simulink model "LD1"  (Simulink 7.9)
settings: Solver=ode3  StartTime=0.0  StopTime=7.0  FixedStep=1e-4  RelTol=1e-3
libraries: dsparch4 x4, simulink x1
settings Model: Creator=user  LastModifiedBy=user

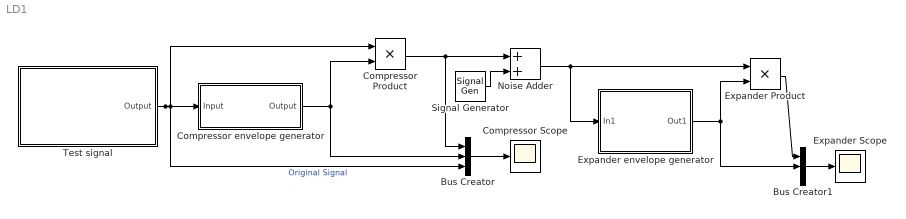
== system LD1 ==
  Bus Creator : BusCreator  Inputs=3
  Bus Creator1 : BusCreator  Inputs=3
  Compressor Product : Product  RndMeth=Zero
  Compressor Scope : Scope
      settings: ShowLegends=on  TimeRange=2.8  YMin=-1.25  YMax=2.25  MaxDataPoints=100000
  "Compressor envelope generator " : Subsystem  mask{S_tr=40, cutoff_frequency=5, dead_zone=0.01}
      mask prompts: S_tr "Scale coefficient"; cutoff_frequency "Filter cutoff (Hz)"; dead_zone "Input signal dead zone level"
      mask Display:
      | Ain = linspace(1, 1e4, 100);
      | Aout = log10(Ain);
      | 
      | plot(Ain, Aout);
  Expander Product : Product  RndMeth=Zero
  Expander Scope : Scope
      settings: ShowLegends=on  TimeRange=2.8  YMin=-1.2  YMax=1.2  MaxDataPoints=100000
  Expander envelope generator : Subsystem  mask{S_tr=40, cutoff_frequency=5, dead_zone=0.01}
      mask prompts: S_tr "Expansion coefficient"; cutoff_frequency "Filter cutoff (Hz)"; dead_zone "Input signal dead zone level"
      mask Display:
      | x = linspace(0,5,1000)
      | y = exp(x)
      | plot(x,y)
  Noise Adder : Sum
  Signal Generator : SignalGenerator  WaveForm=random  Amplitude=0.2
  Test signal : Subsystem  mask{sine_frequency=100, env_time=[0 1 1 2 2 4 4    6    6 7], env_val=[0 0 1 1 0 0 0.5 0.5 0 0]}
      mask prompts: sine_frequency "Sine frequency (Hz)"; env_time "Envelope time points"; env_val "Envelope values"
      mask Display:
      | x = [0 1 1+1e-6 2 2+1e-6 4 4+1e-6 6   6+1e-6 7];
      | y = [0 0 1      1 0      0 0.5    0.5 0      0];
      | x_interp = linspace(0, 7, 100);
      | y_interp = interp1q(x', y', x_interp');
      | 
      | 
      | plot(x_interp, y_interp.*sin(x_interp*10*pi)')
  wires:
  Test signal/1(Output) -> Compressor Product/1, "Compressor envelope generator "/1(Input), Bus Creator/3  "Original Signal"
  "Compressor envelope generator "/1(Output) -> Compressor Product/2, Bus Creator/2
  Bus Creator/1 -> Compressor Scope/1
  Compressor Product/1 -> Bus Creator/1, Noise Adder/1
  Expander envelope generator/1(Out1) -> Expander Product/2, Bus Creator1/2
  Bus Creator1/1 -> Expander Scope/1
  Expander Product/1 -> Bus Creator1/1
  Signal Generator/1 -> Noise Adder/2
  Noise Adder/1 -> Expander Product/1, Expander envelope generator/1(In1)

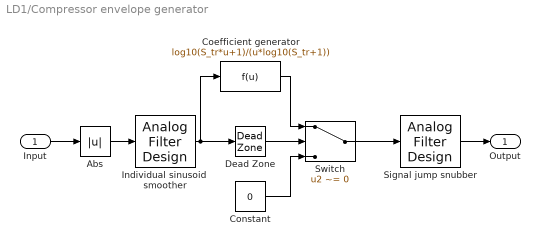
== system LD1/Compressor envelope generator  ==
  Input : Inport
  Abs : Abs
  Coefficient generator : Fcn  Expr=log10(S_tr*u+1)/(u*log10(S_tr+1))
  Constant : Constant  Value=0
  Dead Zone : DeadZone  LowerValue=-dead_zone  UpperValue=dead_zone  SaturateOnIntegerOverflow=on
  Individual sinusoid  smoother : dsparch4/Analog Filter Design  method=Butterworth  filttype=Lowpass  N=1  Wlo=cutoff_frequency*2*pi  Whi=80  Rp=2  Rs=40
  Signal jump snubber : dsparch4/Analog Filter Design  method=Butterworth  filttype=Lowpass  N=1  Wlo=cutoff_frequency/2*2*pi  Whi=80  Rp=2  Rs=40
  Switch : Switch  Criteria=u2 ~= 0
  Output : Outport
  wires:
  Abs/1 -> Individual sinusoid  smoother/1
  Individual sinusoid  smoother/1 -> Coefficient generator/1, Dead Zone/1
  Input/1 -> Abs/1
  Coefficient generator/1 -> Switch/1
  Constant/1 -> Switch/3
  Dead Zone/1 -> Switch/2
  Switch/1 -> Signal jump snubber/1
  Signal jump snubber/1 -> Output/1

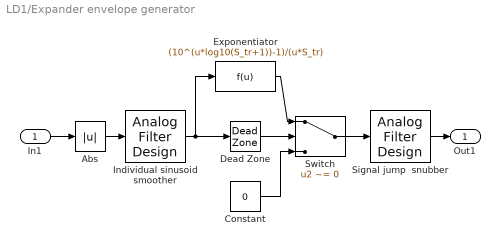
== system LD1/Expander envelope generator ==
  In1 : Inport
  Abs : Abs
  Constant : Constant  Value=0
  Dead Zone : DeadZone  LowerValue=-dead_zone  UpperValue=dead_zone  SaturateOnIntegerOverflow=on
  Exponentiator : Fcn  Expr=(10^(u*log10(S_tr+1))-1)/(u*S_tr)
  Individual sinusoid smoother : dsparch4/Analog Filter Design  method=Butterworth  filttype=Lowpass  N=1  Wlo=cutoff_frequency*2*pi  Whi=80  Rp=2  Rs=40
  Signal jump  snubber : dsparch4/Analog Filter Design  method=Butterworth  filttype=Lowpass  N=1  Wlo=cutoff_frequency/2*2*pi  Whi=80  Rp=2  Rs=40
  Switch : Switch  Criteria=u2 ~= 0
  Out1 : Outport
  wires:
  In1/1 -> Abs/1
  Exponentiator/1 -> Switch/1
  Constant/1 -> Switch/3
  Dead Zone/1 -> Switch/2
  Individual sinusoid smoother/1 -> Dead Zone/1, Exponentiator/1
  Abs/1 -> Individual sinusoid smoother/1
  Switch/1 -> Signal jump  snubber/1
  Signal jump  snubber/1 -> Out1/1

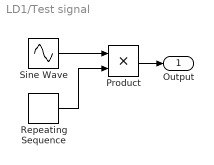
== system LD1/Test signal ==
  Product : Product  RndMeth=Zero
  Repeating Sequence : simulink/Sources/Repeating Sequence  rep_seq_t=env_time  rep_seq_y=env_val
  Sine Wave : Sin  Frequency=sine_frequency*2*pi  SampleTime=0
  Output : Outport
  wires:
  Sine Wave/1 -> Product/1
  Repeating Sequence/1 -> Product/2
  Product/1 -> Output/1
